simulink model "test_nlin_interp"  (R2015a)
settings: Solver=ode1  StartTime=0.0  StopTime=u(end,1)  FixedStep=0.001  RelTol=1e-3
PostLoadFcn:
  | , if any(exist('dsrtsu_mdlpostloadfcn', 'file') == [2, 3, 6]), try dsrtsu_mdlpostloadfcn('Execute', bdroot); catch fprintf('Error in PostLoadFcn (dsrtsu_mdlpostloadfcn) for model "%s":\n %s\n', bdroot, lasterr); end, end,
values from neighbouring files (symbols this model uses):
  c = rectangle('Parent',ax)    [DoublePendulum.m]    (also in init.m = 2.99880047981; interpolate.m = 2.99880047981; plot_17.m = 2.99880047981)
  g = 9.81    [init.m]    (also in interpolate.m; plot_17.m; plot_generic.m)
  T1 = 0.0395    [init.m]    (also in interpolate.m = 0.025; plot_17.m = 0.025; plot_generic.m)
settings Model: DSRTSU_INTERNAL_RTI_VER=360  DSRTSU_INTERNAL_RTI_TYPE=rti1104  CovSFcnEnable=off  Creator=labor  LastModifiedBy=Schuettler
settings DataIOCC: LimitDataPoints=off  SignalLoggingSaveFormat=ModelDataLogs
settings OptimizationCC: BlockReduction=off  OptimizeBlockIOStorage=off  BufferReuse=off  GlobalBufferReuse=off  ExpressionFolding=off  ExpressionDepthLimit=2147483647  LocalBlockOutputs=off  InitFltsAndDblsToZero=on  OptimizeModelRefInitCode=on  LifeSpan=1
settings DebuggingCC: UnderspecifiedInitializationDetection=Classic  MergeDetectMultiDrivingBlocksExec=none  SolverPrmCheckMsg=warning  FcnCallInpInsideContextMsg=UseLocalSettings  StateNameClashWarn=warning
settings HardwareCC: ProdIntDivRoundTo=Zero  ProdEndianess=BigEndian  ProdHWDeviceType=Generic->Custom  TargetIntDivRoundTo=Zero  TargetEndianess=BigEndian  TargetHWDeviceType=Generic->Custom
settings RTWCC: SystemTargetFile=ert.tlc  TemplateMakefile=ert_default_tmf  Description=Embedded Coder
settings CodeAppCC: IgnoreCustomStorageClasses=off
settings ERTTargetCC: ParMdlRefBuildCompliant=on  CompOptLevelCompliant=on  ConcurrentExecutionCompliant=on  ERTFirstTimeCompliant=on  SupportContinuousTime=off  SupportVariableSizeSignals=off  ModelStepFunctionPrototypeControlCompliant=on  CPPClassGenCompliant=on  InlinedParameterPlacement=Hierarchical  ERTCustomFileTemplate=example_file_process.tlc

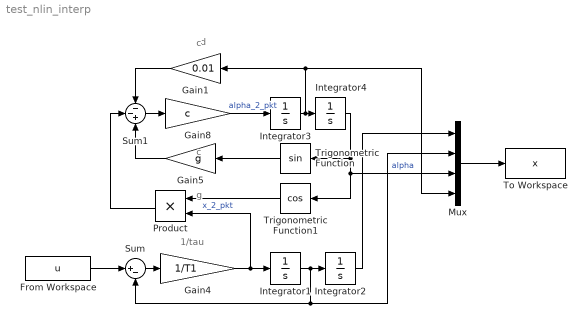
== system test_nlin_interp ==
  note: d
  note: 1/tau
  note: g
  note: c
  note: c
  From Workspace : FromWorkspace  VariableName=u  SampleTime=0
  Gain1 : Gain  Gain=0.01
  Gain4 : Gain  Gain=1/T1
  Gain5 : Gain  Gain=g
  Gain8 : Gain  Gain=c
  Integrator1 : Integrator
  Integrator2 : Integrator
  Integrator3 : Integrator
  Integrator4 : Integrator  InitialCondition=pi
  Mux : Mux
  Product : Product  RndMeth=Zero
  Sum : Sum  Inputs=|+-
  Sum1 : Sum  Inputs=--+
  To Workspace : ToWorkspace  VariableName=x  SampleTime=-1
  Trigonometric Function : Trigonometry
  Trigonometric Function1 : Trigonometry  Operator=cos
  wires:
  Integrator1/1 -> Sum/2, Mux/2, Integrator2/1
  Integrator3/1 -> Mux/4, Gain1/1, Integrator4/1
  Gain4/1 -> Integrator1/1, Product/2  "x_2_pkt"
  Sum/1 -> Gain4/1
  Trigonometric Function1/1 -> Product/1
  Sum1/1 -> Gain8/1
  Gain8/1 -> Integrator3/1  "alpha_2_pkt"
  Integrator4/1 -> Mux/3, Trigonometric Function1/1, Trigonometric Function/1  "alpha"
  Integrator2/1 -> Mux/1
  Trigonometric Function/1 -> Gain5/1
  Gain5/1 -> Sum1/3
  From Workspace/1 -> Sum/1
  Product/1 -> Sum1/2
  Gain1/1 -> Sum1/1
  Mux/1 -> To Workspace/1
